simulink model "pto11_I_menos_PD_SIMU"  (R2017b)
settings: Solver=VariableStepAuto  StartTime=0.0  StopTime=10.0  RelTol=1e-3
settings Model: Creator=Cx001la  LastModifiedBy=Cx001la

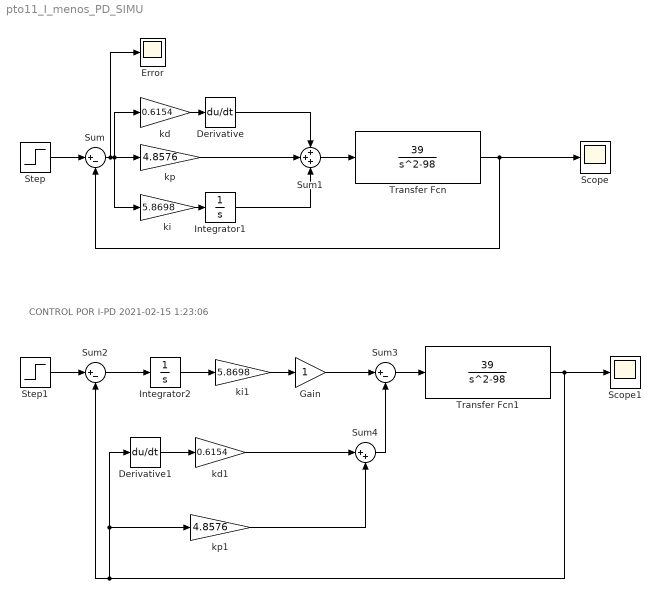
== system pto11_I_menos_PD_SIMU ==
  note: CONTROL POR I-PD 2021-02-15 1:23:06
  Derivative : Derivative
  Derivative1 : Derivative
  Error : Scope
  Gain : Gain
  Integrator1 : Integrator
  Integrator2 : Integrator
  Scope : Scope
  Scope1 : Scope
  Step : Step  Time=0  SampleTime=0
  Step1 : Step  Time=0  SampleTime=0
  Sum : Sum  Inputs=|+-
  Sum1 : Sum  Inputs=+++
  Sum2 : Sum  Inputs=|+-
  Sum3 : Sum  Inputs=|+-
  Sum4 : Sum  Inputs=|++
  Transfer Fcn : TransferFcn  Numerator=[39]  Denominator=[1 0 -98]
  Transfer Fcn1 : TransferFcn  Numerator=[39]  Denominator=[1 0 -98]
  kd : Gain  Gain=0.6154
  kd1 : Gain  Gain=0.6154
  ki : Gain  Gain=5.8698
  ki1 : Gain  Gain=5.8698
  kp : Gain  Gain=4.8576
  kp1 : Gain  Gain=4.8576
  wires:
  Sum/1 -> Error/1, ki/1, kd/1, kp/1
  ki/1 -> Integrator1/1
  kd/1 -> Derivative/1
  Derivative/1 -> Sum1/1
  kp/1 -> Sum1/2
  Integrator1/1 -> Sum1/3
  Sum1/1 -> Transfer Fcn/1
  Transfer Fcn/1 -> Scope/1, Sum/2
  Step/1 -> Sum/1
  Step1/1 -> Sum2/1
  Sum2/1 -> Integrator2/1
  Integrator2/1 -> ki1/1
  Sum4/1 -> Sum3/2
  kd1/1 -> Sum4/1
  Derivative1/1 -> kd1/1
  kp1/1 -> Sum4/2
  Sum3/1 -> Transfer Fcn1/1
  ki1/1 -> Gain/1
  Gain/1 -> Sum3/1
  Transfer Fcn1/1 -> Scope1/1, kp1/1, Derivative1/1, Sum2/2
